simulink model "GroupNavSimulation"  (R2013a)
settings: Solver=ode45  StartTime=0.0  StopTime=10.0  RelTol=1e-3
settings Model: Creator=josh  LastModifiedBy=josh

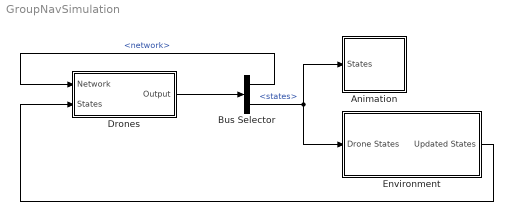
== system GroupNavSimulation ==
  Animation : Subsystem
  Bus Selector : BusSelector  OutputSignals=network,states
  Drones : Subsystem
  Environment : Subsystem
  wires:
  Environment/1(Updated States) -> Drones/2(States)
  Drones/1(Output) -> Bus Selector/1
  Bus Selector/1 -> Drones/1(Network)  "<network>"
  Bus Selector/2 -> Animation/1(States), Environment/1(Drone States)  "<states>"

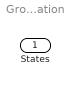
== system GroupNavSimulation/Animation ==
  States : Inport

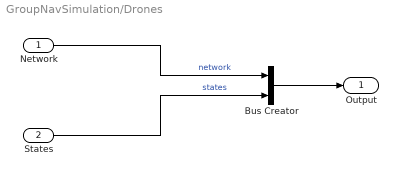
== system GroupNavSimulation/Drones ==
  Network : Inport
  States : Inport  Port=2
  Bus Creator : BusCreator  Inputs=2
  Output : Outport
  wires:
  Network/1 -> Bus Creator/1  "network"
  States/1 -> Bus Creator/2  "states"
  Bus Creator/1 -> Output/1

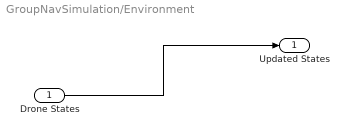
== system GroupNavSimulation/Environment ==
  Drone States : Inport
  Updated States : Outport
  wires:
  Drone States/1 -> Updated States/1
